simulink model "task2_wtch"  (R2024a)
settings: Solver=VariableStepAuto  StartTime=0.0  StopTime=10.0  RelTol=1e-3
settings Model: Creator=sizgr  LastModifiedBy=kit

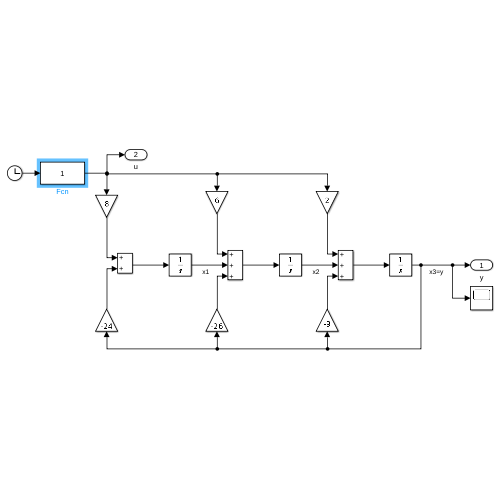
[thumbnail: Simulink's stored preview of the top-level diagram]
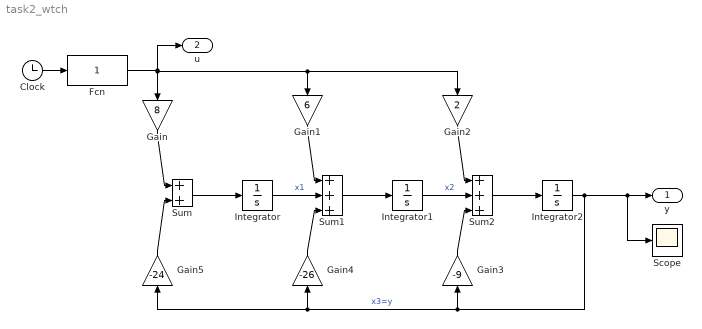
== system task2_wtch ==
  Clock : Clock
  Fcn : Fcn  Expr=1
  Gain : Gain  Gain=8
  Gain1 : Gain  Gain=6
  Gain2 : Gain  Gain=2
  Gain3 : Gain  Gain=-9
  Gain4 : Gain  Gain=-26
  Gain5 : Gain  Gain=-24
  Integrator : Integrator
  Integrator1 : Integrator
  Integrator2 : Integrator
  Scope : Scope
  Sum : Sum
  Sum1 : Sum  Inputs=+++
  Sum2 : Sum  Inputs=+++
  y : Outport
  u : Outport  Port=2
  wires:
  Fcn/1 -> u/1, Gain/1, Gain2/1, Gain1/1
  Gain/1 -> Sum/1
  Sum/1 -> Integrator/1
  Integrator/1 -> Sum1/2  "x1"
  Sum1/1 -> Integrator1/1
  Integrator1/1 -> Sum2/2  "x2"
  Sum2/1 -> Integrator2/1
  Integrator2/1 -> Gain5/1, Gain4/1, Gain3/1, Scope/1, y/1  "x3=y"
  Gain2/1 -> Sum2/1
  Gain1/1 -> Sum1/1
  Gain5/1 -> Sum/2
  Gain4/1 -> Sum1/3
  Gain3/1 -> Sum2/3
  Clock/1 -> Fcn/1
